simulink model "mfcm_hw"  (Simulink 7.1)
settings: Solver=VariableStepDiscrete  StartTime=0.0  StopTime=1200  RelTol=1e-3
undefined symbols (not defined in the file): mimo_setup
libraries: xbsIndex_r4 x42, xbsCopyrightNotice_r4 x1, xrbsComm_r4 x1
settings Model: Creator=alexc  LastModifiedBy=bchan
settings OptimizationCC: InlineInvariantSignals=on
settings DebuggingCC: SaveWithParameterizedLinksMsg=none  SignalResolutionControl=TryResolveAllWithWarning  SolverPrmCheckMsg=none  MultiTaskDSMMsg=warning  MultiTaskCondExecSysMsg=none  StrictBusMsg=None
settings RTWCC: IncludeERTFirstTime=on
settings GRTTargetCC: TargetFcnLib=ansi_tfl_tmw.mat

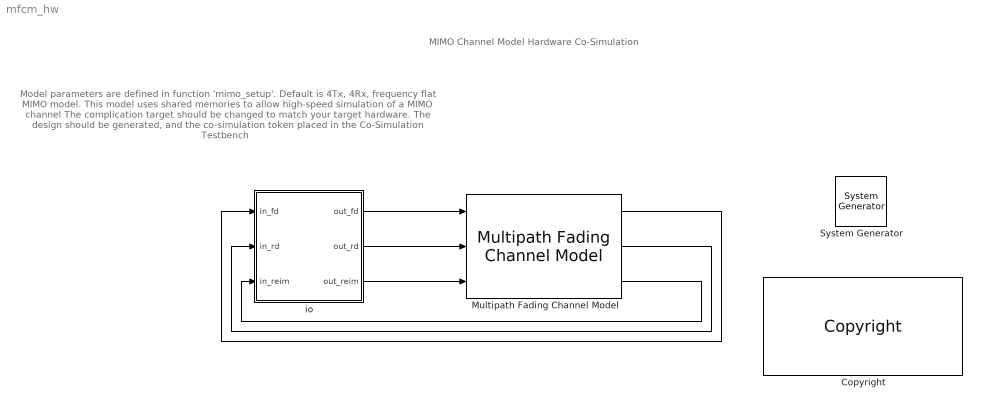
== system mfcm_hw ==
  note: Model parameters are defined in function 'mimo_setup'.
      | Default is 4Tx, 4Rx, frequency flat MIMO model.
      |
      | This model uses shared memories to allow high-speed simulation of a MIMO channel
      | The complication target should be changed to match your target hardware.
      | The design should be generated, and the co-simulation token placed in the Co-Simulation Testbench
  note: MIMO Channel Model Hardware Co-Simulation
  " System Generator" : xbsIndex_r4/ System Generator  Tag=genX  SystemSampleTime=-1  xilinxfamily=virtex5  part=xc5vsx50t  speed=-1  package=ff1136  synthesis_tool=XST  clock_wrapper=Clock Enables  directory=./netlist  testbench=off  simulink_period=1  sysclk_period=10  dcm_input_clock_period=10  incr_netlist=off  trim_vbits=Everywhere in SubSystem  dbl_ovrd=According to Block Masks  core_generation=According to Block Masks  run_coregen=off  deprecated_control=off  eval_field=0  block_type=sysgen
      settings: block_version=11.3
  Copyright : xbsCopyrightNotice_r4/Copyright  copyrighttext="Copyright (c) 2009  by  Xilinx, Inc. All rights reserved.<br><br>This file contains proprietary, confidential information of Xilinx, Inc., is distributed under licensefrom Xilinx, Inc., and may be used, copied and/or disclosed only pursuant to the terms of a valid licenseagreement with Xilinx, Inc. Xilinx hereby grants you a license to use this file solely for design,simulation, implementation and creation of design files limited to Xilinx devices or technologies. Use with non-Xilinx devices or technologies is expressly prohibited and immediately terminates your license unless covered by a separate agreement.<br><br>Xilinx is providing this design, code, or information \"as-is\" solely for use in developing programs and solutions for Xilinx devices, with no obligation on the part of Xilinx to provide support. By providingthis design, code, or information as one possible implementation of this feature, application or standard,Xilinx is making no representation that this implementation is free from any claims of infringement. Youare responsible for obtaining any rights you may require for your implementation. Xilinx expressly disclaimsany warranty whatsoever with respect to the adequacy of the implementation, including but not limited to anywarranties or representations that this implementation is free from claims of infringement, implied warrantiesof merchantability or fitness for a particular purpose.<br><br>Xilinx products are not intended for use in life support appliances, devices, or systems. Use in such applications is expressly prohibited.<br><br>Any modifications that are made to the Source Code are done at the user's sole risk and will be unsupported.<br><br>This copyright and support notice must be retained as part of this text at all times. (c) Copyright 1995-2009 Xilinx, Inc. All rights reserved."  block_type=copyright
      settings: block_version=11.3
  Multipath Fading Channel Model : xrbsComm_r4/Multipath Fading Channel Model  SystemSampleTime=-1  DELAY=mimo_setup('delay')  GAIN=mimo_setup('gain')  RT=mimo_setup('Rt')  RR=mimo_setup('Rr')  SPEC_DATA=mimo_setup('spec_data')  RATE=mimo_setup('rate')  DATAPATH_WIDTH=18  TX_BINPT=17  FADE_BINPT=15  RX_BINPT=15  MAT_BINPT=17  SEED='461AF8228C9F8C92'  block_type=delay
      link override matrix ops/fading_matrix/cg/idft/safe_mac/mfcm_mac: BlockChoice=mfcm_mac_sim
      link override matrix ops/fading_matrix/multiply SCMAT by SCVEC/comp_mac/im_mac/mfcm_mac: BlockChoice=mfcm_mac_sim
      link override matrix ops/fading_matrix/multiply SCMAT by SCVEC/comp_mac/re_mac/mfcm_mac: BlockChoice=mfcm_mac_sim
      link override matrix ops/rx_matrix/multiply SCMAT by SCVEC/comp_mac/im_mac/mfcm_mac: BlockChoice=mfcm_mac_sim
      link override matrix ops/rx_matrix/multiply SCMAT by SCVEC/comp_mac/re_mac/mfcm_mac: BlockChoice=mfcm_mac_sim
      link override matrix ops/tx_matrix/comp_mac/im_mac/mfcm_mac: BlockChoice=mfcm_mac_sim
      link override matrix ops/tx_matrix/comp_mac/re_mac/mfcm_mac: BlockChoice=mfcm_mac_sim
      settings: infoedit=Multipath Fading Channel Model.  block_version=VER_STRING_GOES_HERE
  io : Subsystem  mask{TX_ROWS=mimo_setup('Mt'), TX_WIDTH=18, TX_BINPT=17, RX_ROWS=mimo_setup('Mr'), RX_WIDTH=18, RX_BINPT=15, COLS=1024, TX_PERIOD=mimo_setup('Tmin')}
      mask prompts: TX_ROWS "Tx Vector Size"; TX_WIDTH "Tx Symbol Width"; TX_BINPT "Tx Symbol Binary Point"; RX_ROWS "Rx Vector Size"; RX_WIDTH "Rx Symbol Width"; RX_BINPT "Rx Symbol Binary Point"; COLS "Number of Symbol Vectors"; TX_PERIOD "Input Vector Period"
  wires:
  io/1(out_fd) -> Multipath Fading Channel Model/1
  io/2(out_rd) -> Multipath Fading Channel Model/2
  io/3(out_reim) -> Multipath Fading Channel Model/3
  Multipath Fading Channel Model/3 -> io/3(in_reim)
  Multipath Fading Channel Model/2 -> io/2(in_rd)
  Multipath Fading Channel Model/1 -> io/1(in_fd)

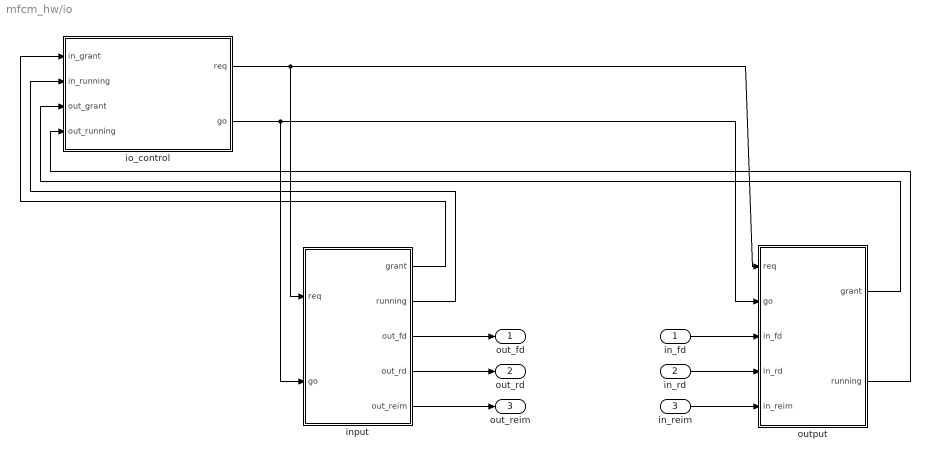
== system mfcm_hw/io ==
  in_fd : Inport  OutDataType=sfix(16)  OutScaling=2^0
  in_rd : Inport  Port=2  OutDataType=sfix(16)  OutScaling=2^0
  in_reim : Inport  Port=3  OutDataType=sfix(16)  OutScaling=2^0
  input : Subsystem  mask{IN_ROWS=TX_ROWS, IN_COLS=COLS, IN_PERIOD=TX_PERIOD, IN_WIDTH=TX_WIDTH, IN_BINPT=TX_BINPT}
      mask prompts: IN_ROWS "Input Rows"; IN_COLS "Input Columns"; IN_PERIOD "Input Vector Period"; IN_WIDTH "Input Width"; IN_BINPT "Input Binary Point"
  io_control : Subsystem
  output : Subsystem  mask{OUT_ROWS=RX_ROWS, OUT_COLS=COLS, OUT_WIDTH=RX_WIDTH, OUT_BINPT=RX_BINPT}
      mask prompts: OUT_ROWS "Output Rows"; OUT_COLS "Output Columns"; OUT_WIDTH "Output Width"; OUT_BINPT "Output Binary Point"
  out_fd : Outport  OutDataType=sfix(16)  OutScaling=2^0
  out_rd : Outport  Port=2  OutDataType=sfix(16)  OutScaling=2^0
  out_reim : Outport  Port=3  OutDataType=sfix(16)  OutScaling=2^0
  wires:
  io_control/1(req) -> input/1(req), output/1(req)
  io_control/2(go) -> input/2(go), output/2(go)
  input/1(grant) -> io_control/1(in_grant)
  output/1(grant) -> io_control/3(out_grant)
  input/2(running) -> io_control/2(in_running)
  output/2(running) -> io_control/4(out_running)
  input/3(out_fd) -> out_fd/1
  in_fd/1 -> output/3(in_fd)
  input/4(out_rd) -> out_rd/1
  in_rd/1 -> output/4(in_rd)
  input/5(out_reim) -> out_reim/1
  in_reim/1 -> output/5(in_reim)

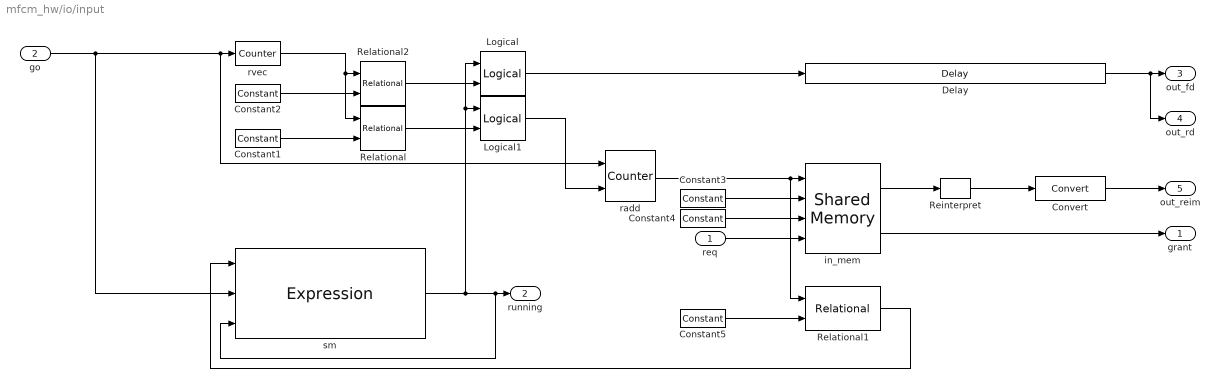
== system mfcm_hw/io/input ==
  req : Inport  OutDataType=sfix(16)  OutScaling=2^0
  go : Inport  Port=2  OutDataType=sfix(16)  OutScaling=2^0
  Constant1 : xbsIndex_r4/Constant  arith_type=Unsigned  const=2*IN_ROWS  n_bits=ceil(log2(IN_PERIOD))  bin_pt=0  explicit_period=off  period=1  equ=P=C  opselect=C  inp2=PCIN>>17  opr=+  inp1=P  carry=CIN  dbl_ovrd=off  block_type=constant
      settings: block_version=VER_STRING_GOES_HERE
  Constant2 : xbsIndex_r4/Constant  arith_type=Unsigned  const=0  n_bits=ceil(log2(IN_PERIOD))  bin_pt=0  explicit_period=off  period=1  equ=P=C  opselect=C  inp2=PCIN>>17  opr=+  inp1=P  carry=CIN  dbl_ovrd=off  block_type=constant
      settings: block_version=VER_STRING_GOES_HERE
  Constant3 : xbsIndex_r4/Constant  arith_type=Signed (2's comp)  const=0  n_bits=32  bin_pt=0  explicit_period=off  period=1  equ=P=C  opselect=C  inp2=PCIN>>17  opr=+  inp1=P  carry=CIN  dbl_ovrd=off  block_type=constant
      settings: block_version=VER_STRING_GOES_HERE
  Constant4 : xbsIndex_r4/Constant  arith_type=Boolean  const=0  n_bits=1  bin_pt=0  explicit_period=off  period=1  equ=P=C  opselect=C  inp2=PCIN>>17  opr=+  inp1=P  carry=CIN  dbl_ovrd=off  block_type=constant
      settings: block_version=VER_STRING_GOES_HERE
  Constant5 : xbsIndex_r4/Constant  arith_type=Unsigned  const=IN_COLS*2*IN_ROWS-1  n_bits=ceil(log2(IN_COLS*2*IN_ROWS))  bin_pt=0  explicit_period=off  period=1  equ=P=C  opselect=C  inp2=PCIN>>17  opr=+  inp1=P  carry=CIN  dbl_ovrd=off  block_type=constant
      settings: block_version=VER_STRING_GOES_HERE
  Convert : xbsIndex_r4/Convert  arith_type="Signed  (2's comp)"  n_bits=TX_WIDTH  bin_pt=TX_BINPT  quantization=Truncate  overflow=Wrap  latency=1  dbl_ovrd=off  pipeline=off  block_type=convert
      settings: infoedit=The input is presented at the output after quantization and overflow effects.<P><P>Hardware notes: Additional hardware is used when rounding or saturation is selected and output width is less than the input width.  block_version=VER_STRING_GOES_HERE
  Delay : xbsIndex_r4/Delay  en=off  latency=2  dbl_ovrd=off  reg_retiming=off  block_type=delay
      settings: infoedit="Delay line having  configurable length.<P><P>Hardware notes: A delay line is a chain, each link of which is an SRL16 followed by a flip-flop. If register retiming is enabled, the delay line is a chain of flip-flops."  block_version=VER_STRING_GOES_HERE
  Logical : xbsIndex_r4/Logical  logical_function=AND  inputs=2  en=off  latency=1  precision=Full  arith_type=Unsigned  n_bits=8  bin_pt=2  align_bp=on  dbl_ovrd=off  block_type=logical
      settings: block_version=VER_STRING_GOES_HERE
  Logical1 : xbsIndex_r4/Logical  logical_function=AND  inputs=2  en=off  latency=1  precision=Full  arith_type=Unsigned  n_bits=8  bin_pt=2  align_bp=on  dbl_ovrd=off  block_type=logical
      settings: block_version=VER_STRING_GOES_HERE
  Reinterpret : xbsIndex_r4/Reinterpret  force_arith_type=on  arith_type="Signed  (2's comp)"  force_bin_pt=on  bin_pt=24  block_type=cast
      settings: infoedit="Changes type of samples without altering their binary representation.<P><P>Hardware notes: In hardware this block costs nothing.<P><P>Example:  Suppose the input is 6 bits wide, signed, with 2 fractional bits, and the output is forced to unsigned with 0 fractional bits.  Then an input of -2.0 (1110.00 in binary 2's complement) becomes an output of 56 (111000 in binary)."  block_version=VER_STRING_GOES_HERE
  Relational : xbsIndex_r4/Relational  mode=a<b  en=off  latency=0  dbl_ovrd=off  block_type=relational
      settings: block_version=VER_STRING_GOES_HERE
  Relational1 : xbsIndex_r4/Relational  mode=a=b  en=off  latency=1  dbl_ovrd=off  block_type=relational
      settings: block_version=VER_STRING_GOES_HERE
  Relational2 : xbsIndex_r4/Relational  mode=a=b  en=off  latency=0  dbl_ovrd=off  block_type=relational
      settings: block_version=VER_STRING_GOES_HERE
  in_mem : xbsIndex_r4/Shared Memory  shared_memory_name='in_mem'  depth=IN_COLS*2*IN_ROWS  ownership=Locally Owned and Initialized  initVector=repmat([1; -1]*sqrt(2)/2,IN_ROWS,IN_COLS)  mutex=Lockable  mode=Read and Write  write_mode=No Read On Write  time_out=1  latency=1  explicit_data_type=off  arith_type="Signed  (2's comp)"  n_bits=32  bin_pt=0  implementation=Block RAM  use_rpm=on  block_type=shmem
      settings: AttributesFormatString=<< %<shared_memory_name> >>  block_version=VER_STRING_GOES_HERE
  radd : xbsIndex_r4/Counter  cnt_type=Free Running  cnt_to=Inf  operation=Up  start_count=0  cnt_by_val=1  arith_type=Unsigned  n_bits=ceil(log2(IN_COLS*2*IN_ROWS))  bin_pt=0  load_pin=off  rst=on  en=on  explicit_period=off  period=1  dbl_ovrd=off  use_behavioral_HDL=off  implementation=Fabric  block_type=counter
      settings: infoedit="Configurable up, down and up/down counter.<P><P>Hardware notes: Free running counters are the least expensive in hardware.  A count limited counter is implemented by combining a counter with a comparator."  block_version=VER_STRING_GOES_HERE
  rvec : xbsIndex_r4/Counter  cnt_type=Count Limited  cnt_to=IN_PERIOD-1  operation=Up  start_count=0  cnt_by_val=1  arith_type=Unsigned  n_bits=ceil(log2(IN_PERIOD))  bin_pt=0  load_pin=off  rst=on  en=off  explicit_period=off  period=1  dbl_ovrd=off  use_behavioral_HDL=off  implementation=Fabric  block_type=counter
      settings: infoedit="Configurable up, down and up/down counter.<P><P>Hardware notes: Free running counters are the least expensive in hardware.  A count limited counter is implemented by combining a counter with a comparator."  block_version=VER_STRING_GOES_HERE
  sm : xbsIndex_r4/Expression  expression=go | (running & ~done)  align_bp=on  en=off  latency=1  precision=Full  arith_type=Unsigned  n_bits=8  bin_pt=2  dbl_ovrd=off  block_type=expr
      settings: block_version=VER_STRING_GOES_HERE
  grant : Outport  OutDataType=sfix(16)  OutScaling=2^0
  running : Outport  Port=2  OutDataType=sfix(16)  OutScaling=2^0
  out_fd : Outport  Port=3  OutDataType=sfix(16)  OutScaling=2^0
  out_rd : Outport  Port=4  OutDataType=sfix(16)  OutScaling=2^0
  out_reim : Outport  Port=5  OutDataType=sfix(16)  OutScaling=2^0
  wires:
  radd/1 -> in_mem/1, Relational1/1
  in_mem/2 -> grant/1
  in_mem/1 -> Reinterpret/1
  Constant2/1 -> Relational2/2
  Constant1/1 -> Relational/2
  go/1 -> rvec/1, radd/1, sm/2
  rvec/1 -> Relational2/1, Relational/1
  Relational2/1 -> Logical/2
  Relational/1 -> Logical1/2
  Logical/1 -> Delay/1
  Logical1/1 -> radd/2
  Delay/1 -> out_fd/1, out_rd/1
  Convert/1 -> out_reim/1
  Relational1/1 -> sm/1
  Constant5/1 -> Relational1/2
  sm/1 -> Logical/1, Logical1/1, running/1, sm/3
  Reinterpret/1 -> Convert/1
  Constant3/1 -> in_mem/2
  Constant4/1 -> in_mem/3
  req/1 -> in_mem/4

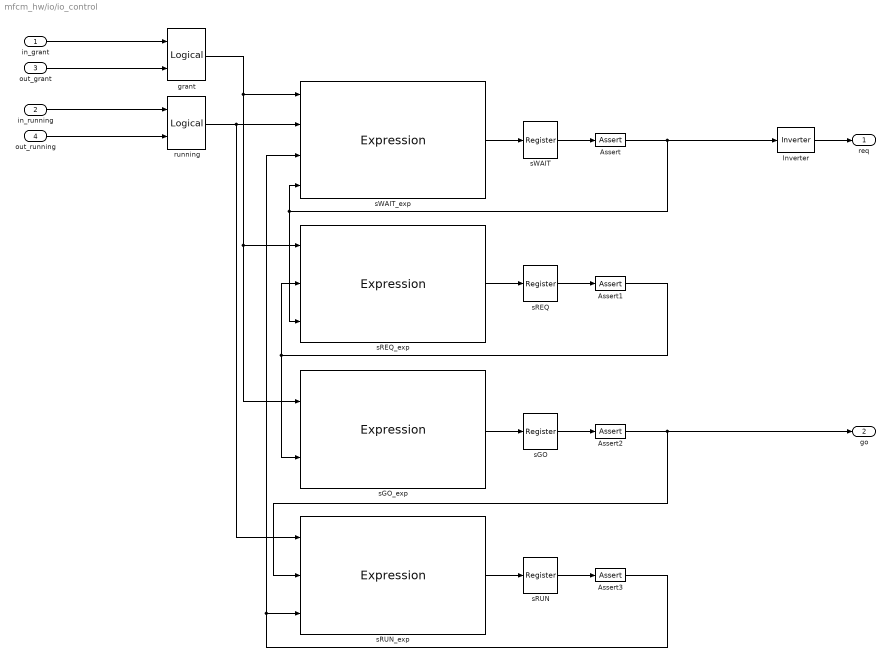
== system mfcm_hw/io/io_control ==
  in_grant : Inport  OutDataType=sfix(16)  OutScaling=2^0
  in_running : Inport  Port=2  OutDataType=sfix(16)  OutScaling=2^0
  out_grant : Inport  Port=3  OutDataType=sfix(16)  OutScaling=2^0
  out_running : Inport  Port=4  OutDataType=sfix(16)  OutScaling=2^0
  Assert{,1..3} (4 alike) : xbsIndex_r4/Assert  assert_type=on  type_source=Explicitly  arith_type=Boolean  n_bits=8  bin_pt=2  assert_rate=on  rate_source=Explicitly  period=1  output_port=on  block_type=assert
      settings: infoedit=Asserts a user-defined sample rate and/or type on a signal.  block_version=VER_STRING_GOES_HERE
  Inverter : xbsIndex_r4/Inverter  en=off  latency=0  dbl_ovrd=off  block_type=inv
      settings: block_version=VER_STRING_GOES_HERE
  grant : xbsIndex_r4/Logical  logical_function=AND  inputs=2  en=off  latency=0  precision=Full  arith_type=Unsigned  n_bits=8  bin_pt=2  align_bp=on  dbl_ovrd=off  block_type=logical
      settings: block_version=VER_STRING_GOES_HERE
  running : xbsIndex_r4/Logical  logical_function=OR  inputs=2  en=off  latency=0  precision=Full  arith_type=Unsigned  n_bits=8  bin_pt=2  align_bp=on  dbl_ovrd=off  block_type=logical
      settings: block_version=VER_STRING_GOES_HERE
  sGO : xbsIndex_r4/Register  init=0  rst=off  en=off  dbl_ovrd=off  block_type=register
      settings: block_version=VER_STRING_GOES_HERE
  sGO_exp : xbsIndex_r4/Expression  expression=(sREQ & grant)  align_bp=on  en=off  latency=0  precision=Full  arith_type=Unsigned  n_bits=8  bin_pt=2  dbl_ovrd=off  block_type=expr
      settings: block_version=VER_STRING_GOES_HERE
  sREQ : xbsIndex_r4/Register  init=0  rst=off  en=off  dbl_ovrd=off  block_type=register
      settings: block_version=VER_STRING_GOES_HERE
  sREQ_exp : xbsIndex_r4/Expression  expression=(sWAIT & ~grant) | (sREQ & ~grant)  align_bp=on  en=off  latency=0  precision=Full  arith_type=Unsigned  n_bits=8  bin_pt=2  dbl_ovrd=off  block_type=expr
      settings: block_version=VER_STRING_GOES_HERE
  sRUN : xbsIndex_r4/Register  init=0  rst=off  en=off  dbl_ovrd=off  block_type=register
      settings: block_version=VER_STRING_GOES_HERE
  sRUN_exp : xbsIndex_r4/Expression  expression=sGO | (sRUN & running)  align_bp=on  en=off  latency=0  precision=Full  arith_type=Unsigned  n_bits=8  bin_pt=2  dbl_ovrd=off  block_type=expr
      settings: block_version=VER_STRING_GOES_HERE
  sWAIT : xbsIndex_r4/Register  init=1  rst=off  en=off  dbl_ovrd=off  block_type=register
      settings: block_version=VER_STRING_GOES_HERE
  sWAIT_exp : xbsIndex_r4/Expression  expression=(sRUN & ~running) | (sWAIT & grant)  align_bp=on  en=off  latency=0  precision=Full  arith_type=Unsigned  n_bits=8  bin_pt=2  dbl_ovrd=off  block_type=expr
      settings: block_version=VER_STRING_GOES_HERE
  req : Outport  OutDataType=sfix(16)  OutScaling=2^0
  go : Outport  Port=2  OutDataType=sfix(16)  OutScaling=2^0
  wires:
  sWAIT_exp/1 -> sWAIT/1
  sWAIT/1 -> Assert/1
  in_grant/1 -> grant/1
  out_grant/1 -> grant/2
  in_running/1 -> running/1
  out_running/1 -> running/2
  grant/1 -> sWAIT_exp/1, sREQ_exp/1, sGO_exp/1
  running/1 -> sWAIT_exp/2, sRUN_exp/1
  sREQ_exp/1 -> sREQ/1
  sREQ/1 -> Assert1/1
  sGO_exp/1 -> sGO/1
  sGO/1 -> Assert2/1
  sRUN_exp/1 -> sRUN/1
  sRUN/1 -> Assert3/1
  Inverter/1 -> req/1
  Assert/1 -> sWAIT_exp/4, sREQ_exp/3, Inverter/1
  Assert1/1 -> sREQ_exp/2, sGO_exp/2
  Assert2/1 -> go/1, sRUN_exp/2
  Assert3/1 -> sRUN_exp/3, sWAIT_exp/3

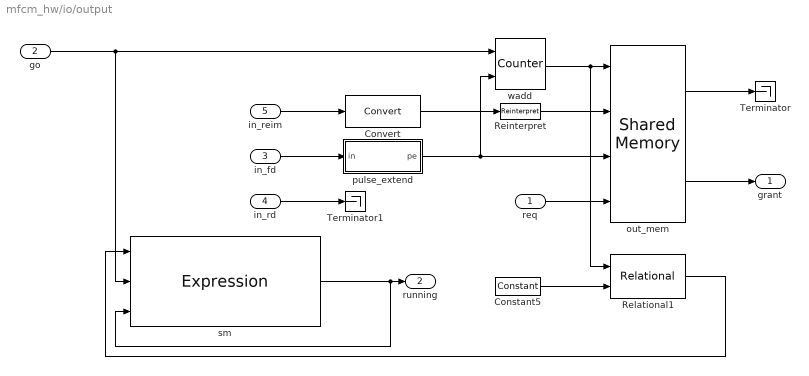
== system mfcm_hw/io/output ==
  req : Inport  OutDataType=sfix(16)  OutScaling=2^0
  go : Inport  Port=2  OutDataType=sfix(16)  OutScaling=2^0
  in_fd : Inport  Port=3  OutDataType=sfix(16)  OutScaling=2^0
  in_rd : Inport  Port=4  OutDataType=sfix(16)  OutScaling=2^0
  in_reim : Inport  Port=5  OutDataType=sfix(16)  OutScaling=2^0
  Constant5 : xbsIndex_r4/Constant  arith_type=Unsigned  const=OUT_COLS*2*OUT_ROWS-1  n_bits=ceil(log2(OUT_COLS*2*OUT_ROWS))  bin_pt=0  explicit_period=off  period=1  equ=P=C  opselect=C  inp2=PCIN>>17  opr=+  inp1=P  carry=CIN  dbl_ovrd=off  block_type=constant
      settings: block_version=VER_STRING_GOES_HERE
  Convert : xbsIndex_r4/Convert  arith_type="Signed  (2's comp)"  n_bits=32  bin_pt=24  quantization=Truncate  overflow=Wrap  latency=0  dbl_ovrd=off  pipeline=off  block_type=convert
      settings: infoedit=The input is presented at the output after quantization and overflow effects.<P><P>Hardware notes: Additional hardware is used when rounding or saturation is selected and output width is less than the input width.  block_version=VER_STRING_GOES_HERE
  Reinterpret : xbsIndex_r4/Reinterpret  force_arith_type=on  arith_type="Signed  (2's comp)"  force_bin_pt=on  bin_pt=0  block_type=cast
      settings: infoedit="Changes type of samples without altering their binary representation.<P><P>Hardware notes: In hardware this block costs nothing.<P><P>Example:  Suppose the input is 6 bits wide, signed, with 2 fractional bits, and the output is forced to unsigned with 0 fractional bits.  Then an input of -2.0 (1110.00 in binary 2's complement) becomes an output of 56 (111000 in binary)."  block_version=VER_STRING_GOES_HERE
  Relational1 : xbsIndex_r4/Relational  mode=a=b  en=off  latency=1  dbl_ovrd=off  block_type=relational
      settings: block_version=VER_STRING_GOES_HERE
  Terminator : Terminator
  Terminator1 : Terminator
  out_mem : xbsIndex_r4/Shared Memory  shared_memory_name='out_mem'  depth=OUT_COLS*2*OUT_ROWS  ownership=Locally Owned and Initialized  initVector=0  mutex=Lockable  mode=Read and Write  write_mode=No Read On Write  time_out=1  latency=1  explicit_data_type=off  arith_type="Signed  (2's comp)"  n_bits=32  bin_pt=0  implementation=Block RAM  use_rpm=on  block_type=shmem
      settings: AttributesFormatString=<< %<shared_memory_name> >>  block_version=VER_STRING_GOES_HERE
  pulse_extend : Subsystem
  sm : xbsIndex_r4/Expression  expression=go | (running & ~done)  align_bp=on  en=off  latency=1  precision=Full  arith_type=Unsigned  n_bits=8  bin_pt=2  dbl_ovrd=off  block_type=expr
      settings: block_version=VER_STRING_GOES_HERE
  wadd : xbsIndex_r4/Counter  cnt_type=Free Running  cnt_to=Inf  operation=Up  start_count=0  cnt_by_val=1  arith_type=Unsigned  n_bits=ceil(log2(OUT_COLS*2*OUT_ROWS))  bin_pt=0  load_pin=off  rst=on  en=on  explicit_period=off  period=1  dbl_ovrd=off  use_behavioral_HDL=off  implementation=Fabric  block_type=counter
      settings: infoedit="Configurable up, down and up/down counter.<P><P>Hardware notes: Free running counters are the least expensive in hardware.  A count limited counter is implemented by combining a counter with a comparator."  block_version=VER_STRING_GOES_HERE
  grant : Outport  OutDataType=sfix(16)  OutScaling=2^0
  running : Outport  Port=2  OutDataType=sfix(16)  OutScaling=2^0
  wires:
  sm/1 -> running/1, sm/3
  go/1 -> wadd/1, sm/2
  req/1 -> out_mem/4
  wadd/1 -> out_mem/1, Relational1/1
  in_reim/1 -> Convert/1
  in_rd/1 -> Terminator1/1
  in_fd/1 -> pulse_extend/1(in)
  pulse_extend/1(pe) -> wadd/2, out_mem/3
  Constant5/1 -> Relational1/2
  Relational1/1 -> sm/1
  Convert/1 -> Reinterpret/1
  Reinterpret/1 -> out_mem/2
  out_mem/2 -> grant/1
  out_mem/1 -> Terminator/1

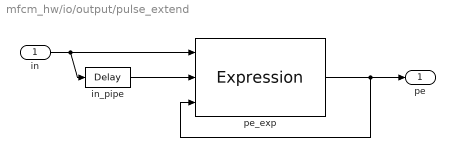
== system mfcm_hw/io/output/pulse_extend ==
  in : Inport  OutDataType=sfix(16)  OutScaling=2^0
  in_pipe : xbsIndex_r4/Delay  en=off  latency=2*OUT_ROWS  dbl_ovrd=off  reg_retiming=off  block_type=delay
      settings: infoedit="Delay line having  configurable length.<P><P>Hardware notes: A delay line is a chain, each link of which is an SRL16 followed by a flip-flop. If register retiming is enabled, the delay line is a chain of flip-flops."  block_version=VER_STRING_GOES_HERE
  pe_exp : xbsIndex_r4/Expression  expression=in0 | (pe & ~inz)  align_bp=on  en=off  latency=1  precision=Full  arith_type=Unsigned  n_bits=8  bin_pt=2  dbl_ovrd=off  block_type=expr
      settings: block_version=VER_STRING_GOES_HERE
  pe : Outport  OutDataType=sfix(16)  OutScaling=2^0
  wires:
  in_pipe/1 -> pe_exp/2
  pe_exp/1 -> pe_exp/3, pe/1
  in/1 -> in_pipe/1, pe_exp/1
